simulink model "planner_contral"  (R2023b)
settings: Solver=FixedStepAuto  StartTime=0  StopTime=inf  FixedStep=0.001  RelTol=1e-3
undefined symbols (not defined in the file): aubr, c_factor, cf, cr, iniObsHeading1, iniObsHeading2, iniObsPos1, iniObsPos2, KD_PID_distance, KD_PID_speed, KI_PID_distance, KI_PID_speed, KP_PID_distance, KP_PID_speed, la, lb, LQR_K1, LQR_K2, LQR_K3, LQR_K4, m, rack_displacement, refInfo_obs1, refInfo_obs2, right_wheel_ground, rightWaypoints, tablebr, vubr, vx_break_point
libraries: Solver_SF x1
(part 1 of 8)
settings Model: NumberOfSteps=100  Creator=Ally  LastModifiedBy=pc
settings DebuggingCC: UnconnectedInputMsg=warning  UnconnectedOutputMsg=warning  UnconnectedLineMsg=warning  UnderSpecifiedDimensionMsg=warning
settings ModelReferenceCC: EnableRefExpFcnMdlSchedulingChecks=on
settings RTWCC: DLArmComputeVersion=19.05

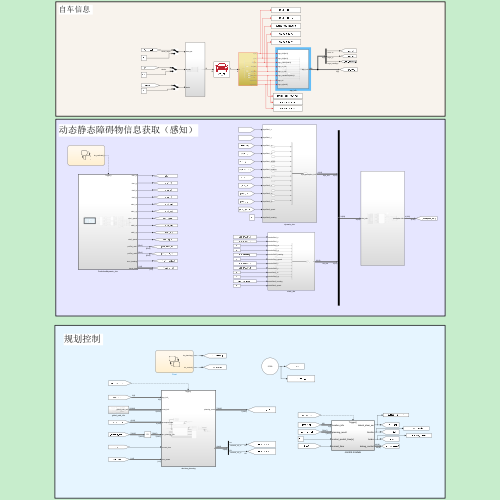
[thumbnail: Simulink's stored preview of the top-level diagram]
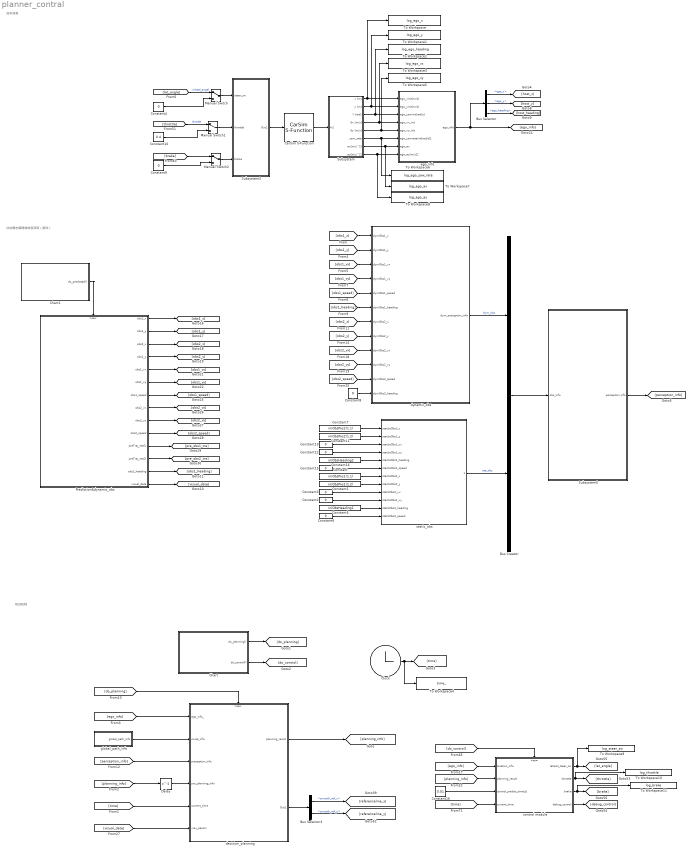
== system planner_contral ==
  note: 动态静态障碍物信息获取（感知）
  note: 规划控制
  note: 自车信息
  Bus Creator : BusCreator  Inputs=2
  Bus Selector : BusSelector  OutputSignals=ego_x,ego_y,ego_heading
  Bus Selector3 : BusSelector  OutputSignals=smooth_ref_x,smooth_ref_y
  CarSim S-Function : Solver_SF/CarSim S-Function  Priority=1  SIMFILE=simfile.sim  Run_RTs=off  vs_state_ind=Run  StopMode_ind=Vehicle Model
  Chart : Stateflow chart  TreatAsAtomicUnit=on
  Chart1 : Stateflow chart  TreatAsAtomicUnit=on
  Clock : Clock
  Constant : Constant  Value=iniObsPos1(1,1)
  Constant1 : Constant  Value=iniObsPos1(1,2)
  Constant10 : Constant  Value=0.4
  Constant11 : Constant  Value=iniObsPos2(1,2)
  Constant{2..4,6,8..9,12..13,15} (9 alike) : Constant  Value=0
  Constant14 : Constant  Value=iniObsHeading2
  Constant16 : Constant  Value=0.01
  Constant5 : Constant  Value=iniObsHeading1
  Constant7 : Constant  Value=iniObsPos2(1,1)
  Delay : Delay  DelayLength=1
  Manual Switch : ManualSwitch
  Manual Switch1 : ManualSwitch
  Manual Switch2 : ManualSwitch
  Prediction&dynamic_obs : Subsystem
  Subsystem : Subsystem
  Subsystem3 : Subsystem
  Subsystem5 : Subsystem
  To Workspace : ToWorkspace  VariableName=log_ego_x  SaveFormat=Timeseries  SampleTime=-1
  To Workspace1 : ToWorkspace  VariableName=log_ego_y  SaveFormat=Timeseries  SampleTime=-1
  To Workspace10 : ToWorkspace  VariableName=log_throttle  SampleTime=-1
  To Workspace11 : ToWorkspace  VariableName=log_brake  SampleTime=-1
  To Workspace2 : ToWorkspace  VariableName=log_ego_heading  SaveFormat=Timeseries  SampleTime=-1
  To Workspace3 : ToWorkspace  VariableName=log_ego_vx  SaveFormat=Timeseries  SampleTime=-1
  To Workspace4 : ToWorkspace  VariableName=time_  SaveFormat=Timeseries  SampleTime=-1
  To Workspace5 : ToWorkspace  VariableName=log_ego_vy  SaveFormat=Timeseries  SampleTime=-1
  To Workspace6 : ToWorkspace  VariableName=log_ego_yaw_rate  SaveFormat=Timeseries  SampleTime=-1
  To Workspace7 : ToWorkspace  VariableName=log_ego_ax  SaveFormat=Timeseries  SampleTime=-1
  To Workspace8 : ToWorkspace  VariableName=log_ego_ay  SaveFormat=Timeseries  SampleTime=-1
  To Workspace9 : ToWorkspace  VariableName=log_steer_sw  SampleTime=-1
  control module : Subsystem
  decision_planning : Subsystem
  dynamic_obs : Subsystem
  ego_info : Subsystem
  global_path_info : Subsystem
  static_obs : Subsystem
  wires:
  Chart/2(do_control()) -> [do_control]
  Clock/1 -> [time], To Workspace4/1
  Chart/1(do_planning()) -> [do_planning]
  [do_planning] -> decision_planning/Trigger
  global_path_info/1(global_path_info) -> decision_planning/2(route_info)
  [time] -> decision_planning/5(current_time)
  [planning_info] -> Delay/1
  [ego_info] -> decision_planning/1(ego_info_)
  Delay/1 -> decision_planning/4(pro_planning_info)
  decision_planning/2(Out1) -> Bus Selector3/1
  Bus Selector3/1 -> [referenceline_x]  "<smooth_ref_x>"
  Bus Selector3/2 -> [referenceline_y]  "<smooth_ref_y>"
  decision_planning/1(planning_result) -> [planning_info]
  control module/2(throttle) -> To Workspace10/1, [throttle]
  [do_control] -> control module/Trigger
  [time] -> control module/4(current_time)
  Constant16/1 -> control module/3(control_predict_time[s])
  control module/4(debug_control) -> [debug_control]
  control module/1(lateral_steer_sw) -> To Workspace9/1, [lat_angle]
  control module/3(brake) -> To Workspace11/1, [brake]
  [ego_info] -> control module/1(location_info)
  [planning_info] -> control module/2(planning_result)
  Subsystem/2(y [m]) -> To Workspace1/1, ego_info/2(ego_yinit[m/s])
  Subsystem/4(dx [m/s]) -> To Workspace3/1, ego_info/4(ego_vx_init)
  Subsystem/5(dy [m/s]) -> To Workspace5/1, ego_info/5(ego_vy_init)
  Subsystem/3(Y [rad]) -> To Workspace2/1, ego_info/3(ego_yawinit[rad/s])
  Subsystem/6(yaw_rate) -> To Workspace6/1, ego_info/6(ego_yawrateinit[rad/s]1)
  Subsystem/7(ax[m/s^2]) -> To Workspace7/1, ego_info/7(ego_ax)
  Subsystem/8(ay[m/s^2]) -> To Workspace8/1, ego_info/8(ego_ay[m/s2])
  ego_info/1(ego_info) -> [ego_info], Bus Selector/1
  Constant4/1 -> Manual Switch/2
  Constant9/1 -> Manual Switch2/2
  [brake] -> Manual Switch2/1
  [throttle] -> Manual Switch1/1  "throtle"
  [lat_angle] -> Manual Switch/1  "wheel_angel"
  Manual Switch/1 -> Subsystem3/1(steer_sw)
  Manual Switch2/1 -> Subsystem3/3(brake)
  Subsystem/1(x [m]) -> To Workspace/1, ego_info/1(ego_xinit[m/s])
  CarSim S-Function/1 -> Subsystem/1(In1)
  Bus Selector/1 -> [host_x]  "<ego_x>"
  Bus Selector/2 -> [host_y]  "<ego_y>"
  Bus Selector/3 -> [host_heading]  "<ego_heading>"
  Constant10/1 -> Manual Switch1/2
  Manual Switch1/1 -> Subsystem3/2(throttle)
  Prediction&dynamic_obs/1(obs1_x) -> [obs1_x]
  Prediction&dynamic_obs/2(obs1_y) -> [obs1_y]
  Prediction&dynamic_obs/4(obs2_y) -> [obs2_y]
  Prediction&dynamic_obs/5(obs1_vx) -> [obs1_vx]
  Prediction&dynamic_obs/6(obs1_vy) -> [obs1_vy]
  Prediction&dynamic_obs/7(obs1_speed) -> [obs1_speed]
  Prediction&dynamic_obs/8(obs2_vx) -> [obs2_vx]
  Prediction&dynamic_obs/9(obs2_vy) -> [obs2_vy]
  Prediction&dynamic_obs/10(obs2_speed) -> [obs2_speed]
  Prediction&dynamic_obs/11(preTraj_real1) -> [pre_obs1_tra]
  Prediction&dynamic_obs/12(preTraj_real2) -> [pre_obs2_tra]
  [obs1_speed] -> dynamic_obs/5(dymObs1_speed)
  [obs1_x] -> dynamic_obs/1(dymObs1_x)
  [obs1_heading] -> dynamic_obs/6(dymObs1_heading)
  [obs1_y] -> dynamic_obs/2(dymObs1_y)
  [obs1_vy] -> dynamic_obs/4(dymObs1_vy)
  static_obs/1(s) -> Bus Creator/2  "sta_obs"
  [obs1_vx] -> dynamic_obs/3(dymObs1_vx)
  dynamic_obs/1(dym_preception_info) -> Bus Creator/1  "dym_obs"
  Bus Creator/1 -> Subsystem5/1(obs_info)
  Prediction&dynamic_obs/3(obs2_x) -> [obs2_x]
  Prediction&dynamic_obs/13(obs1_heading) -> [obs1_heading]
  [visual_date] -> decision_planning/6(visu_param)
  Chart1/1(do_predicted()) -> Prediction&dynamic_obs/Trigger
  [obs2_vy] -> dynamic_obs/10(dymObs2_vy)
  [obs2_x] -> dynamic_obs/7(dymObs2_x)
  [obs2_vx] -> dynamic_obs/9(dymObs2_vx)
  [obs2_y] -> dynamic_obs/8(dymObs2_y)
  [obs2_speed] -> dynamic_obs/11(dymObs2_speed)
  Constant8/1 -> dynamic_obs/12(dymObs2_heading)
  Subsystem3/1(Out1) -> CarSim S-Function/1
  Prediction&dynamic_obs/14(visual_data) -> [visual_date]
  Subsystem5/1(perception info) -> [perception_info]
  [perception_info] -> decision_planning/3(preception_info)
  Constant15/1 -> static_obs/6(stacticObs1_speed)
  Constant13/1 -> static_obs/3(stacticObs1_vx)
  Constant7/1 -> static_obs/1(stacticObs1_x)
  Constant11/1 -> static_obs/2(stacticObs1_y)
  Constant12/1 -> static_obs/4(stacticObs1_vy)
  Constant14/1 -> static_obs/5(stacticObs1_heading)
  Constant/1 -> static_obs/7(stacticObs2_x)
  Constant1/1 -> static_obs/8(stacticObs2_y)
  Constant3/1 -> static_obs/9(staticObs2_vx)
  Constant2/1 -> static_obs/10(stacticObs2_vy)
  Constant5/1 -> static_obs/11(staticObs2_heading)
  Constant6/1 -> static_obs/12(staticObs2_speed)

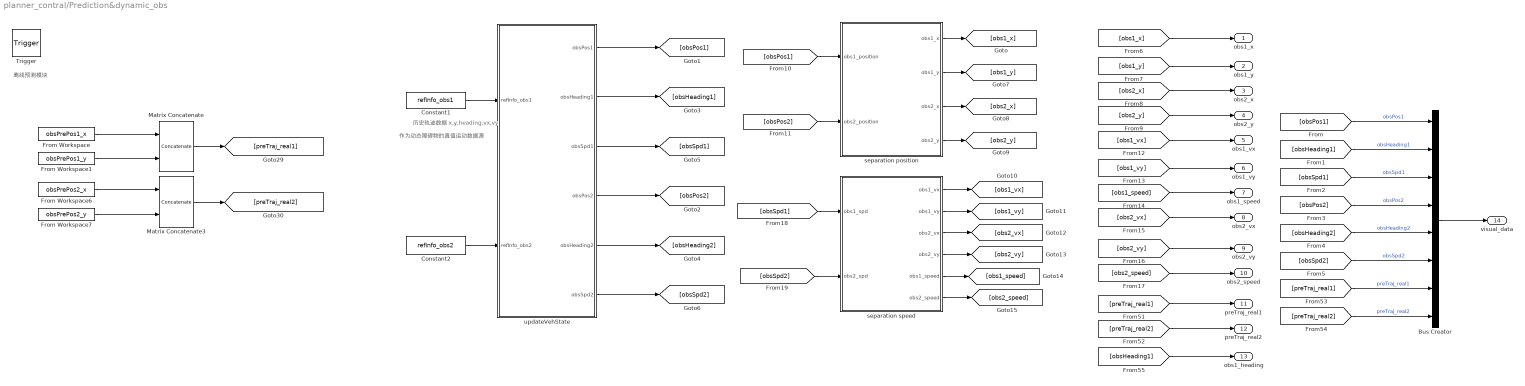
== system planner_contral/Prediction&dynamic_obs ==
  note: 作为动态障碍物的真值运动数据源
  note: 历史轨迹数据
      | x,y,heading,vx,vy
  note: 离线预测模块
  Trigger : TriggerPort  TriggerType=function-call  VariantControl=(inherit)  PortDimensions=1
  Bus Creator : BusCreator  Inputs=8
  Constant1 : Constant  Value=refInfo_obs1
  Constant2 : Constant  Value=refInfo_obs2
  From Workspace : FromWorkspace  VariableName=obsPrePos1_x  SampleTime=-1
  From Workspace1 : FromWorkspace  VariableName=obsPrePos1_y  SampleTime=-1
  From Workspace6 : FromWorkspace  VariableName=obsPrePos2_x  SampleTime=-1
  From Workspace7 : FromWorkspace  VariableName=obsPrePos2_y  SampleTime=-1
  Matrix Concatenate : Concatenate  Mode=Multidimensional array  ConcatenateDimension=2
  Matrix Concatenate3 : Concatenate  Mode=Multidimensional array  ConcatenateDimension=2
  separation position : MATLAB Function  TreatAsAtomicUnit=on
  separation speed : MATLAB Function  TreatAsAtomicUnit=on
  updateVehState : MATLAB Function  TreatAsAtomicUnit=on
  obs1_x : Outport
  obs1_y : Outport  Port=2
  obs2_x : Outport  Port=3
  obs2_y : Outport  Port=4
  obs1_vx : Outport  Port=5
  obs1_vy : Outport  Port=6
  obs1_speed : Outport  Port=7
  obs2_vx : Outport  Port=8
  obs2_vy : Outport  Port=9
  obs2_speed : Outport  Port=10
  preTraj_real1 : Outport  Port=11
  preTraj_real2 : Outport  Port=12
  obs1_heading : Outport  Port=13
  visual_data : Outport  Port=14
  wires:
  updateVehState/5(obsHeading2) -> [obsHeading2]
  Constant2/1 -> updateVehState/2(refInfo_obs2)
  updateVehState/4(obsPos2) -> [obsPos2]
  updateVehState/6(obsSpd2) -> [obsSpd2]
  updateVehState/3(obsSpd1) -> [obsSpd1]
  Constant1/1 -> updateVehState/1(refInfo_obs1)
  Matrix Concatenate/1 -> [preTraj_real1]
  From Workspace7/1 -> Matrix Concatenate3/2
  From Workspace/1 -> Matrix Concatenate/1
  From Workspace1/1 -> Matrix Concatenate/2
  Matrix Concatenate3/1 -> [preTraj_real2]
  [obs1_x] -> obs1_x/1
  [obs1_y] -> obs1_y/1
  [obs2_x] -> obs2_x/1
  [obs2_y] -> obs2_y/1
  [obsPos1] -> separation position/1(obs1_position)
  [obsPos2] -> separation position/2(obs2_position)
  separation position/1(obs1_x) -> [obs1_x]
  separation position/2(obs1_y) -> [obs1_y]
  separation position/3(obs2_x) -> [obs2_x]
  separation position/4(obs2_y) -> [obs2_y]
  [obs2_vx] -> obs2_vx/1
  [obs1_vx] -> obs1_vx/1
  [obs1_vy] -> obs1_vy/1
  [obs1_speed] -> obs1_speed/1
  [obs2_vy] -> obs2_vy/1
  [obs2_speed] -> obs2_speed/1
  separation speed/3(obs2_vx) -> [obs2_vx]
  separation speed/4(obs2_vy) -> [obs2_vy]
  separation speed/2(obs1_vy) -> [obs1_vy]
  separation speed/1(obs1_vx) -> [obs1_vx]
  [obsSpd2] -> separation speed/2(obs2_spd)
  [obsSpd1] -> separation speed/1(obs1_spd)
  separation speed/5(obs1_speed) -> [obs1_speed]
  separation speed/6(obs2_speed) -> [obs2_speed]
  From Workspace6/1 -> Matrix Concatenate3/1
  [preTraj_real1] -> preTraj_real1/1
  [preTraj_real2] -> preTraj_real2/1
  [obsPos1] -> Bus Creator/1  "obsPos1"
  [obsHeading1] -> Bus Creator/2  "obsHeading1"
  [obsSpd1] -> Bus Creator/3  "obsSpd1"
  [obsPos2] -> Bus Creator/4  "obsPos2"
  [obsHeading2] -> Bus Creator/5  "obsHeading2"
  [obsSpd2] -> Bus Creator/6  "obsSpd2"
  [preTraj_real1] -> Bus Creator/7  "preTraj_real1"
  [preTraj_real2] -> Bus Creator/8  "preTraj_real2"
  Bus Creator/1 -> visual_data/1
  [obsHeading1] -> obs1_heading/1
  updateVehState/1(obsPos1) -> [obsPos1]
  updateVehState/2(obsHeading1) -> [obsHeading1]

== system planner_contral/Subsystem ==
  In1 : Inport
  D2R : Gain  Gain=pi/180
  D2R1 : Gain  Gain=pi/180
  Demux : Demux  Outputs=[2 1 2 3]
  Demux1 : Demux  Outputs=2
  Demux2 : Demux  Outputs=2
  Demux4 : Demux  Outputs=3
  Gain : Gain  Gain=9.8
  Gain1 : Gain  Gain=9.8
  km|h_to_m|s : Gain  Gain=1/3.6
  x [m] : Outport
  y [m] : Outport  Port=2
  Y [rad] : Outport  Port=3
  dx [m/s] : Outport  Port=4
  dy [m/s] : Outport  Port=5
  yaw_rate : Outport  Port=6
  ax[m/s^2] : Outport  Port=7
  ay[m/s^2] : Outport  Port=8
  wires:
  In1/1 -> Demux/1
  Demux1/2 -> y [m]/1
  Demux2/1 -> dx [m/s]/1
  Demux4/2 -> Gain/1
  Demux2/2 -> dy [m/s]/1
  Demux/1 -> Demux1/1
  Demux/2 -> D2R/1
  Demux4/3 -> Gain1/1
  Demux1/1 -> x [m]/1
  Demux/3 -> km|h_to_m|s/1
  km|h_to_m|s/1 -> Demux2/1
  Gain1/1 -> ay[m/s^2]/1
  D2R/1 -> Y [rad]/1
  Gain/1 -> ax[m/s^2]/1
  Demux/4 -> Demux4/1
  Demux4/1 -> D2R1/1
  D2R1/1 -> yaw_rate/1

== system planner_contral/Subsystem3 ==
  steer_sw : Inport
  throttle : Inport  Port=2
  brake : Inport  Port=3
  Constant : Constant  Value=zeros(12,1)
  Constant17 : Constant  Value=ones(8,1)*0.9
  Mux1 : Mux  Inputs=[1 1 1 12 8]
  Out1 : Outport
  wires:
  Constant/1 -> Mux1/4
  Mux1/1 -> Out1/1
  brake/1 -> Mux1/3
  steer_sw/1 -> Mux1/1
  throttle/1 -> Mux1/2
  Constant17/1 -> Mux1/5

== system planner_contral/Subsystem5 ==
  note: 障碍物状态整理 / 打包 / 标准接口输出
  note: 最多 32 个障碍物的
      | 位置 x
      | 位置 y
      | 速度大小 v
      | 速度方向 heading
  obs_info : Inport
  Bus Creator : BusCreator  Inputs=4
  Bus Selector2 : BusSelector  OutputSignals=dym_obs.dymObs1_x,dym_obs.dymObs1_y,dym_obs.dymObs1_vx,dym_obs.dymObs1_vy,dym_obs.dymObs1_speed,dym_obs.dymObs1_heading,dym_obs.dymObs2_x,dym_obs.dymObs2_y,dym_obs.dymObs2_vx,dym_obs.dymObs2_vy,dym_obs.dymObs2_speed,dym_obs.dymObs2_heading,sta_obs.stacticObs1_x,sta_obs.stacticObs1_y,sta_obs.stacticObs1_heading,sta_obs.stacticObs1_speed,sta_obs.stacticObs2_x,sta_obs.stacticObs2_y,sta_obs.staticObs2_heading,sta_obs.staticObs2_speed
  packaging : MATLAB Function  TreatAsAtomicUnit=on
  perception info : Outport
  wires:
  Bus Selector2/9 -> [dynamic_obs2_vx]  "<dymObs2_vx>"
  Bus Selector2/7 -> [dynamic_obs2_x]  "<dymObs2_x>"
  Bus Selector2/12 -> [dynamic_obs2_heading]  "<dymObs2_heading>"
  Bus Selector2/5 -> [dynamic_obs1_speed]  "<dymObs1_speed>"
  Bus Selector2/4 -> [dynamic_obs1_vy]  "<dymObs1_vy>"
  Bus Selector2/15 -> [staticobs1_heading]  "<stacticObs1_heading>"
  [staticobs1_heading] -> packaging/11(stactic_obs1_heading)
  [dynamic_obs1_speed] -> packaging/4(dynamic_obs1_speed)
  [staticobs1_speed] -> packaging/12(stactic_obs1_speed)
  [staticobs1_x] -> packaging/9(stactic_obs1_x)
  Bus Selector2/14 -> [staticobs1_y]  "<stacticObs1_y>"
  [dynamic_obs1_heading] -> packaging/3(dynamic_obs1_heading)
  [staticobs1_y] -> packaging/10(stactic_obs1_y)
  [dynamic_obs1_y] -> packaging/2(dynamic_obs1_y)
  obs_info/1 -> Bus Selector2/1
  [dynamic_obs1_x] -> packaging/1(dynamic_obs1_x)
  Bus Selector2/10 -> [dynamic_obs2_vy]  "<dymObs2_vy>"
  Bus Selector2/2 -> [dynamic_obs1_y]  "<dymObs1_y>"
  Bus Selector2/8 -> [dynamic_obs2_y]  "<dymObs2_y>"
  Bus Selector2/1 -> [dynamic_obs1_x]  "<dymObs1_x>"
  Bus Selector2/3 -> [dynamic_obs1_vx]  "<dymObs1_vx>"
  Bus Selector2/16 -> [staticobs1_speed]  "<stacticObs1_speed>"
  Bus Selector2/13 -> [staticobs1_x]  "<stacticObs1_x>"
  Bus Selector2/11 -> [dynamic_obs2_speed]  "<dymObs2_speed>"
  Bus Selector2/6 -> [dynamic_obs1_heading]  "<dymObs1_heading>"
  [obs_heading_set_gcs] -> Bus Creator/4  "obs_heading_set_gcs"
  [obs_x_set_gcs] -> Bus Creator/1  "obs_x_set_gcs"
  [obs_velocity_set_gcs] -> Bus Creator/3  "obs_velocity_set_gcs"
  Bus Creator/1 -> perception info/1
  [obs_y_set_gcs] -> Bus Creator/2  "obs_y_set_gcs"
  packaging/1(obs_x_set_gcs) -> [obs_x_set_gcs]
  packaging/2(obs_y_set_gcs) -> [obs_y_set_gcs]
  packaging/3(obs_velocity_set_gcs) -> [obs_velocity_set_gcs]
  packaging/4(obs_heading_set_gcs) -> [obs_heading_set_gcs]
  Bus Selector2/17 -> [staticobs2_x]  "<stacticObs2_x>"
  Bus Selector2/18 -> [staticobs2_y]  "<stacticObs2_y>"
  Bus Selector2/19 -> [staticobs2_heading]  "<staticObs2_heading>"
  Bus Selector2/20 -> [staticobs2_speed]  "<staticObs2_speed>"
  [dynamic_obs2_x] -> packaging/5(dynamic_obs2_x)
  [dynamic_obs2_y] -> packaging/6(dynamic_obs2_y)
  [dynamic_obs2_heading] -> packaging/7(dynamic_obs2_heading)
  [dynamic_obs2_speed] -> packaging/8(dynamic_obs2_speed)
  [staticobs2_x] -> packaging/13(stactic_obs2_x)
  [staticobs2_y] -> packaging/14(stactic_obs2_y)
  [staticobs2_heading] -> packaging/15(stactic_obs2_heading)
  [staticobs2_speed] -> packaging/16(stactic_obs2_speed)

== system planner_contral/control module ==
  location_info : Inport
  planning_result : Inport  Port=2
  control_predict_time[s] : Inport  Port=3
  current_time : Inport  Port=4
  Trigger : TriggerPort  TriggerType=function-call  VariantControl=Variant  PortDimensions=1
  Bus Selector : BusSelector  OutputSignals=trajectory_x_gcs,trajectory_y_gcs,trajectory_heading_gcs,trajectory_kappa_gcs,trajectory_speed_gcs,trajectory_accel_gcs,trajectory_time_gcs
  Bus Selector1 : BusSelector  OutputSignals=ego_x,ego_y,ego_heading,ego_vx,ego_vy,ego_yaw_rate,ego_speed
  MATLAB Function : MATLAB Function  TreatAsAtomicUnit=on
  control main : Subsystem
  lateral_steer_sw : Outport
  throttle : Outport  Port=2
  brake : Outport  Port=3
  debug_control : Outport  Port=4
  wires:
  Bus Selector1/5 -> control main/5(host_vy[m/s])  "<ego_vy>"
  Bus Selector1/4 -> control main/4(host_vx[m/s])  "<ego_vx>"
  Bus Selector1/2 -> control main/2(host_y[m])  "<ego_y>"
  Bus Selector1/7 -> control main/7(host_speed[m/s])  "<ego_speed>"
  control main/2(throttle) -> throttle/1
  Bus Selector1/1 -> control main/1(host_x[m])  "<ego_x>"
  Bus Selector1/6 -> control main/6(host_yawrate[rad/s])  "<ego_yaw_rate>"
  Bus Selector1/3 -> control main/3(host_heading_xy[rad])  "<ego_heading>"
  location_info/1 -> Bus Selector1/1
  control_predict_time[s]/1 -> control main/14(control_predict_time[s])
  control main/4(debug_control) -> debug_control/1
  control main/1(lateral_steer_sw) -> lateral_steer_sw/1
  control main/3(brake) -> brake/1
  MATLAB Function/6(ar) -> control main/13(accelerate_desire[m/s^2])
  MATLAB Function/5(vr) -> control main/12(speed_desire[m/s])
  MATLAB Function/4(kappar) -> control main/11(kappar_desire[m^-1])
  MATLAB Function/3(thetar) -> control main/10(thetar_desire[rad])  "desire_yaw"
  MATLAB Function/2(yr) -> control main/9(yr_desire[m])
  MATLAB Function/1(xr) -> control main/8(xr_desire[m])
  current_time/1 -> MATLAB Function/8(current_time)
  planning_result/1 -> Bus Selector/1
  Bus Selector/1 -> [trajecotory_x]  "<trajectory_x_gcs>"
  Bus Selector/2 -> [trajecotory_y]  "<trajectory_y_gcs>"
  Bus Selector/3 -> [trajecotory_heading]  "<trajectory_heading_gcs>"
  Bus Selector/4 -> [trajecotory_kappa]  "<trajectory_kappa_gcs>"
  Bus Selector/5 -> [trajecotory_speed]  "<trajectory_speed_gcs>"
  Bus Selector/6 -> [trajecotory_accel]  "<trajectory_accel_gcs>"
  Bus Selector/7 -> [trajecotory_time]  "<trajectory_time_gcs>"
  [trajecotory_time] -> MATLAB Function/7(trajectory_time)
  [trajecotory_accel] -> MATLAB Function/6(trajectory_accel)
  [trajecotory_speed] -> MATLAB Function/5(trajectory_speed)
  [trajecotory_heading] -> MATLAB Function/3(trajectory_heading)
  [trajecotory_y] -> MATLAB Function/2(trajectory_y)
  [trajecotory_x] -> MATLAB Function/1(trajectory_x)
  [trajecotory_kappa] -> MATLAB Function/4(trajectory_kappa)

== system planner_contral/decision_planning ==
  note: 全局路径 → 局部参考线（给规划用）
  ego_info_ : Inport
  route_info : Inport  Port=2
  preception_info : Inport  Port=3
  pro_planning_info : Inport  Port=4
  current_time : Inport  Port=5
  visu_param : Inport  Port=6
  Trigger : TriggerPort  TriggerType=function-call  VariantControl=(inherit)  PortDimensions=1
  Bus Selector : BusSelector  OutputSignals=ego_x,ego_y,ego_heading
  Bus Selector1 : BusSelector  OutputSignals=smooth_ref_x,smooth_ref_y
  Bus Selector3 : BusSelector  OutputSignals=trajectory_x_gcs,trajectory_y_gcs
  EMplanner : Subsystem
  Visual : Subsystem
  referenceline provider : Subsystem
  planning_result : Outport
  Out1 : Outport  Port=2
  wires:
  referenceline provider/1(referenceline_info) -> [debug_referenceline_info_], [referenceline_info_]
  route_info/1 -> referenceline provider/2(route_info)
  ego_info_/1 -> EMplanner/2(location_info), referenceline provider/1(ego_info), Bus Selector/1
  preception_info/1 -> EMplanner/3(perception info)
  [planning_result] -> planning_result/1
  [referenceline_info_] -> Bus Selector1/1, Out1/1
  Bus Selector/1 -> [host_x]  "<ego_x>"
  Bus Selector/2 -> [host_y]  "<ego_y>"
  Bus Selector/3 -> [host_heading]  "<ego_heading>"
  Bus Selector1/1 -> [referenceline_x]  "<smooth_ref_x>"
  Bus Selector1/2 -> [referenceline_y]  "<smooth_ref_y>"
  EMplanner/1(EM Planner result) -> Bus Selector3/1, [planning_result]
  Bus Selector3/1 -> [trajectory_x]  "<trajectory_x_gcs>"
  Bus Selector3/2 -> [trajectory_y]  "<trajectory_y_gcs>"
  pro_planning_info/1 -> EMplanner/4(pre_planning_info)
  current_time/1 -> EMplanner/5(current_time)
  visu_param/1 -> Visual/3(visu_param), EMplanner/6(visual_data)
  EMplanner/2(plot_visual) -> Visual/1(plot_visual)
  EMplanner/3(tra_ref_info) -> Visual/2(tra_ref)
  [referenceline_info_] -> EMplanner/1(referenceline_info)

== system planner_contral/dynamic_obs ==
  dymObs1_x : Inport
  dymObs1_y : Inport  Port=2
  dymObs1_vx : Inport  Port=3
  dymObs1_vy : Inport  Port=4
  dymObs1_speed : Inport  Port=5
  dymObs1_heading : Inport  Port=6
  dymObs2_x : Inport  Port=7
  dymObs2_y : Inport  Port=8
  dymObs2_vx : Inport  Port=9
  dymObs2_vy : Inport  Port=10
  dymObs2_speed : Inport  Port=11
  dymObs2_heading : Inport  Port=12
  Bus Creator : BusCreator  Inputs=12
  dym_preception_info : Outport
  wires:
  dymObs2_y/1 -> Bus Creator/8  "dymObs2_y"
  dymObs2_vx/1 -> Bus Creator/9  "dymObs2_vx"
  dymObs2_heading/1 -> Bus Creator/12  "dymObs2_heading"
  dymObs2_x/1 -> Bus Creator/7  "dymObs2_x"
  dymObs2_vy/1 -> Bus Creator/10  "dymObs2_vy"
  dymObs1_speed/1 -> Bus Creator/5  "dymObs1_speed"
  dymObs2_speed/1 -> Bus Creator/11  "dymObs2_speed"
  Bus Creator/1 -> dym_preception_info/1
  dymObs1_heading/1 -> Bus Creator/6  "dymObs1_heading"
  dymObs1_vy/1 -> Bus Creator/4  "dymObs1_vy"
  dymObs1_vx/1 -> Bus Creator/3  "dymObs1_vx"
  dymObs1_y/1 -> Bus Creator/2  "dymObs1_y"
  dymObs1_x/1 -> Bus Creator/1  "dymObs1_x"

== system planner_contral/ego_info ==
  ego_xinit[m/s] : Inport
  ego_yinit[m/s] : Inport  Port=2
  ego_yawinit[rad/s] : Inport  Port=3
  ego_vx_init : Inport  Port=4
  ego_vy_init : Inport  Port=5
  ego_yawrateinit[rad/s]1 : Inport  Port=6
  ego_ax : Inport  Port=7
  ego_ay[m/s2] : Inport  Port=8
  Bus Creator : BusCreator  Inputs=9
  MATLAB Function1 : MATLAB Function  TreatAsAtomicUnit=on
  ego_info : Outport
  wires:
  Bus Creator/1 -> ego_info/1
  ego_xinit[m/s]/1 -> Bus Creator/1  "ego_x"
  ego_yinit[m/s]/1 -> Bus Creator/2  "ego_y"
  ego_vy_init/1 -> MATLAB Function1/2(vy), Bus Creator/5  "ego_vy"
  ego_ax/1 -> Bus Creator/8  "ego_ax"
  ego_ay[m/s2]/1 -> Bus Creator/9  "ego_ay"
  ego_vx_init/1 -> Bus Creator/4, MATLAB Function1/1(vx)  "ego_vx"
  ego_yawinit[rad/s]/1 -> Bus Creator/3  "ego_heading"
  ego_yawrateinit[rad/s]1/1 -> Bus Creator/6  "ego_yaw_rate"
  MATLAB Function1/1(y) -> Bus Creator/7  "ego_speed"

== system planner_contral/global_path_info ==
  Bus Creator : BusCreator  Inputs=2
  Constant : Constant  Value=rightWaypoints
  Separation trajectory : MATLAB Function  TreatAsAtomicUnit=on
  global_path_info : Outport
  wires:
  Constant/1 -> Separation trajectory/1(global_xy)
  Separation trajectory/1(global_x_) -> [global_path_x]
  Separation trajectory/2(global_y_) -> [global_path_y]
  [global_path_x] -> Bus Creator/1  "global_path_x"
  [global_path_y] -> Bus Creator/2  "global_path_y"
  Bus Creator/1 -> global_path_info/1

== system planner_contral/static_obs ==
  note: static_obs
  stacticObs1_x : Inport
  stacticObs1_y : Inport  Port=2
  stacticObs1_vx : Inport  Port=3
  stacticObs1_vy : Inport  Port=4
  stacticObs1_heading : Inport  Port=5
  stacticObs1_speed : Inport  Port=6
  stacticObs2_x : Inport  Port=7
  stacticObs2_y : Inport  Port=8
  staticObs2_vx : Inport  Port=9
  stacticObs2_vy : Inport  Port=10
  staticObs2_heading : Inport  Port=11
  staticObs2_speed : Inport  Port=12
  Bus Creator : BusCreator  Inputs=12
  s : Outport
  wires:
  stacticObs1_x/1 -> Bus Creator/1  "stacticObs1_x"
  stacticObs1_y/1 -> Bus Creator/2  "stacticObs1_y"
  stacticObs1_vx/1 -> Bus Creator/3  "stacticObs1_vx"
  stacticObs1_vy/1 -> Bus Creator/4  "stacticObs1_vy"
  stacticObs1_heading/1 -> Bus Creator/5  "stacticObs1_heading"
  Bus Creator/1 -> s/1
  stacticObs1_speed/1 -> Bus Creator/6  "stacticObs1_speed"
  stacticObs2_x/1 -> Bus Creator/7  "stacticObs2_x"
  stacticObs2_y/1 -> Bus Creator/8  "stacticObs2_y"
  staticObs2_vx/1 -> Bus Creator/9  "staticObs2_vx"
  stacticObs2_vy/1 -> Bus Creator/10  "stacticObs2_vy"
  staticObs2_heading/1 -> Bus Creator/11  "staticObs2_heading"
  staticObs2_speed/1 -> Bus Creator/12  "staticObs2_speed"

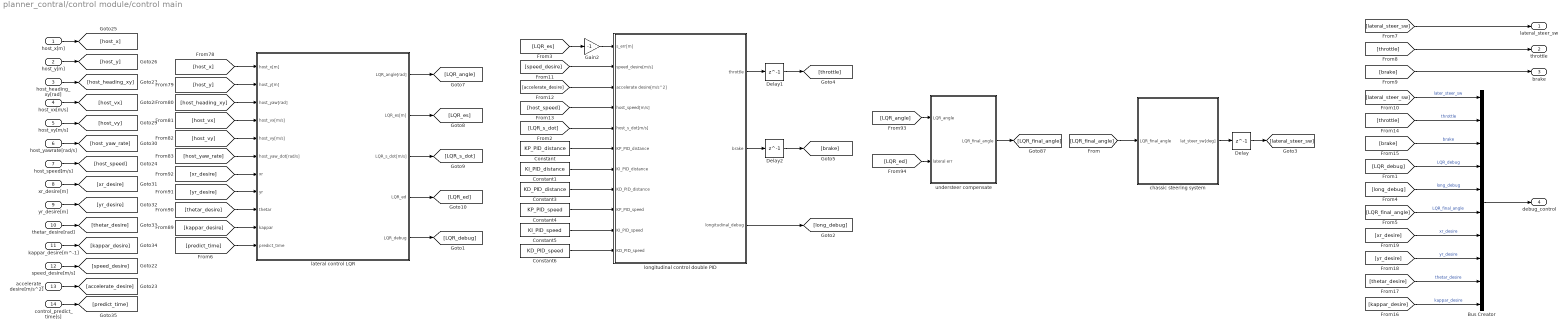
== system planner_contral/control module/control main ==
  host_x[m] : Inport
  host_y[m] : Inport  Port=2
  host_heading_xy[rad] : Inport  Port=3
  host_vx[m/s] : Inport  Port=4
  host_vy[m/s] : Inport  Port=5
  host_yawrate[rad/s] : Inport  Port=6
  host_speed[m/s] : Inport  Port=7
  xr_desire[m] : Inport  Port=8
  yr_desire[m] : Inport  Port=9
  thetar_desire[rad] : Inport  Port=10
  kappar_desire[m^-1] : Inport  Port=11
  speed_desire[m/s] : Inport  Port=12
  accelerate_desire[m/s^2] : Inport  Port=13
  control_predict_time[s] : Inport  Port=14
  Bus Creator : BusCreator  Inputs=10
  Constant : Constant  Value=KP_PID_distance
  Constant1 : Constant  Value=KI_PID_distance
  Constant3 : Constant  Value=KD_PID_distance
  Constant4 : Constant  Value=KP_PID_speed
  Constant5 : Constant  Value=KI_PID_speed
  Constant6 : Constant  Value=KD_PID_speed
  Delay : Delay  DelayLength=1
  Delay1 : Delay  DelayLength=1
  Delay2 : Delay  DelayLength=1
  Gain2 : Gain  Gain=-1
  chassic steering system : Subsystem
  lateral control LQR : Subsystem
  longitudinal control double PID : Subsystem
  understeer compensate : Subsystem
  lateral_steer_sw : Outport
  throttle : Outport  Port=2
  brake : Outport  Port=3
  debug_control : Outport  Port=4
  wires:
  host_x[m]/1 -> [host_x]
  understeer compensate/1(LQR_final_angle) -> [LQR_final_angle]
  lateral control LQR/1(LQR_angle[rad]) -> [LQR_angle]
  [host_vx] -> lateral control LQR/4(host_vx[m/s])
  thetar_desire[rad]/1 -> [thetar_desire]
  Constant1/1 -> longitudinal control double PID/7(KI_PID_distance)
  [accelerate_desire] -> longitudinal control double PID/3(accelerate desire[m/s^2])
  [host_x] -> lateral control LQR/1(host_x[m])
  [xr_desire] -> lateral control LQR/7(xr)
  accelerate_desire[m/s^2]/1 -> [accelerate_desire]
  [host_y] -> lateral control LQR/2(host_y[m])
  [LQR_s_dot] -> longitudinal control double PID/5(host_s_dot[m/s])
  [yr_desire] -> lateral control LQR/8(yr)
  [LQR_angle] -> understeer compensate/1(LQR_angle)
  xr_desire[m]/1 -> [xr_desire]
  [host_vy] -> lateral control LQR/5(host_vy[m/s])
  host_heading_xy[rad]/1 -> [host_heading_xy]
  [LQR_ed] -> understeer compensate/2(lateral err)
  Constant/1 -> longitudinal control double PID/6(KP_PID_distance)
  Constant3/1 -> longitudinal control double PID/8(KD_PID_distance)
  Constant5/1 -> longitudinal control double PID/10(KI_PID_speed)
  Constant4/1 -> longitudinal control double PID/9(KP_PID_speed)
  [host_speed] -> longitudinal control double PID/4(host_speed[m/s])
  [predict_time] -> lateral control LQR/11(predict_time)
  host_vx[m/s]/1 -> [host_vx]
  [speed_desire] -> longitudinal control double PID/2(speed_desire[m/s])
  lateral control LQR/4(LQR_ed) -> [LQR_ed]
  [thetar_desire] -> lateral control LQR/9(thetar)
  [host_heading_xy] -> lateral control LQR/3(host_yaw[rad])
  [kappar_desire] -> lateral control LQR/10(kappar)
  host_yawrate[rad/s]/1 -> [host_yaw_rate]
  kappar_desire[m^-1]/1 -> [kappar_desire]
  yr_desire[m]/1 -> [yr_desire]
  [host_yaw_rate] -> lateral control LQR/6(host_yaw_dot[rad/s])
  host_y[m]/1 -> [host_y]
  host_vy[m/s]/1 -> [host_vy]
  host_speed[m/s]/1 -> [host_speed]
  control_predict_time[s]/1 -> [predict_time]
  speed_desire[m/s]/1 -> [speed_desire]
  Constant6/1 -> longitudinal control double PID/11(KD_PID_speed)
  Gain2/1 -> longitudinal control double PID/1(s_err[m])
  [LQR_es] -> Gain2/1
  [LQR_final_angle] -> chassic steering system/1(LQR_final_angle)
  chassic steering system/1(lat_steer_sw[deg]) -> Delay/1
  longitudinal control double PID/1(throttle) -> Delay1/1
  longitudinal control double PID/2(brake) -> Delay2/1
  lateral control LQR/5(LQR_debug) -> [LQR_debug]
  longitudinal control double PID/3(longitudinal_debug) -> [long_debug]
  Delay/1 -> [lateral_steer_sw]
  Delay1/1 -> [throttle]
  Delay2/1 -> [brake]
  [lateral_steer_sw] -> lateral_steer_sw/1
  [throttle] -> throttle/1
  [brake] -> brake/1
  [lateral_steer_sw] -> Bus Creator/1  "later_steer_sw"
  [throttle] -> Bus Creator/2  "throttle"
  [brake] -> Bus Creator/3  "brake"
  [LQR_debug] -> Bus Creator/4  "LQR_debug"
  [long_debug] -> Bus Creator/5  "long_debug"
  [LQR_final_angle] -> Bus Creator/6  "LQR_final_angle"
  Bus Creator/1 -> debug_control/1
  [xr_desire] -> Bus Creator/7  "xr_desire"
  [yr_desire] -> Bus Creator/8  "yr_desire"
  [thetar_desire] -> Bus Creator/9  "thetar_desire"
  [kappar_desire] -> Bus Creator/10  "kappar_desire"
  lateral control LQR/3(LQR_s_dot[m/s]) -> [LQR_s_dot]
  lateral control LQR/2(LQR_es[m]) -> [LQR_es]
